simulink model "switch_statement"  (R2021a)
settings: Solver=VariableStepAuto  StartTime=0.0  StopTime=10.0  RelTol=1e-3
settings Model: Creator=Acer  LastModifiedBy=Acer

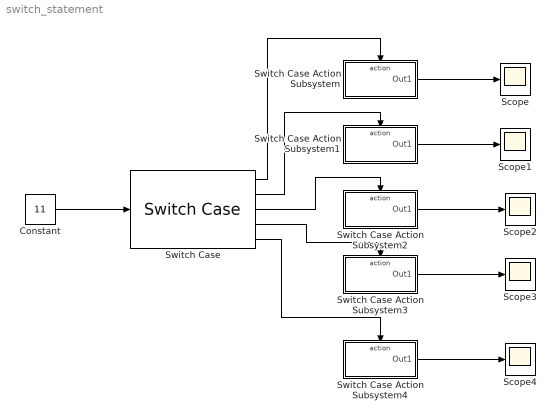
== system switch_statement ==
  Constant : Constant  Value=11
  Scope{,1..4} (5 alike) : Scope
  Switch Case : SwitchCase  CaseConditions={1,[2 3],6,8}
  Switch Case Action Subsystem : Subsystem  TreatAsAtomicUnit=on
  Switch Case Action Subsystem1 : Subsystem  TreatAsAtomicUnit=on
  Switch Case Action Subsystem2 : Subsystem  TreatAsAtomicUnit=on
  Switch Case Action Subsystem3 : Subsystem  TreatAsAtomicUnit=on
  Switch Case Action Subsystem4 : Subsystem  TreatAsAtomicUnit=on
  wires:
  Constant/1 -> Switch Case/1
  Switch Case/3 -> Switch Case Action Subsystem2/Action
  Switch Case/2 -> Switch Case Action Subsystem1/Action
  Switch Case/1 -> Switch Case Action Subsystem/Action
  Switch Case/4 -> Switch Case Action Subsystem3/Action
  Switch Case/5 -> Switch Case Action Subsystem4/Action
  Switch Case Action Subsystem4/1(Out1) -> Scope4/1
  Switch Case Action Subsystem3/1(Out1) -> Scope3/1
  Switch Case Action Subsystem2/1(Out1) -> Scope2/1
  Switch Case Action Subsystem1/1(Out1) -> Scope1/1
  Switch Case Action Subsystem/1(Out1) -> Scope/1

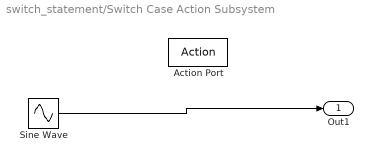
== system switch_statement/Switch Case Action Subsystem ==
  Action Port : ActionPort  ActionPortLabel=case [ 1 ]:
  Sine Wave : Sin  SampleTime=0
  Out1 : Outport
  wires:
  Sine Wave/1 -> Out1/1

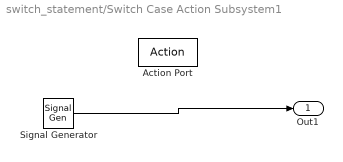
== system switch_statement/Switch Case Action Subsystem1 ==
  Action Port : ActionPort  ActionPortLabel=case [ 2 3 ]:
  Signal Generator : SignalGenerator  WaveForm=sawtooth  Units=rad/sec
  Out1 : Outport
  wires:
  Signal Generator/1 -> Out1/1

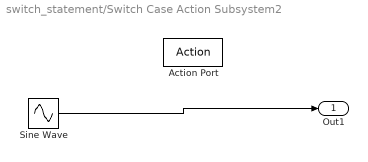
== system switch_statement/Switch Case Action Subsystem2 ==
  Action Port : ActionPort  ActionPortLabel=case [ 6 ]:
  Sine Wave : Sin  Phase=pi/2  SampleTime=0
  Out1 : Outport
  wires:
  Sine Wave/1 -> Out1/1

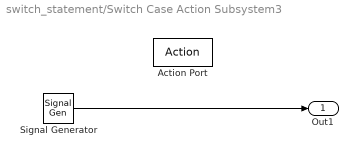
== system switch_statement/Switch Case Action Subsystem3 ==
  Action Port : ActionPort  ActionPortLabel=case [ 8 ]:
  Signal Generator : SignalGenerator  WaveForm=square  Units=rad/sec
  Out1 : Outport
  wires:
  Signal Generator/1 -> Out1/1

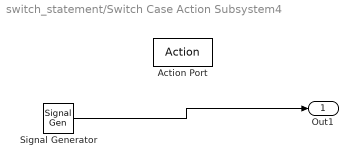
== system switch_statement/Switch Case Action Subsystem4 ==
  Action Port : ActionPort  ActionPortLabel=default:
  Signal Generator : SignalGenerator  WaveForm=random  Units=rad/sec
  Out1 : Outport
  wires:
  Signal Generator/1 -> Out1/1
